simulink model "EarlyReturn12_2018a"  (R2018a)
settings: Solver=VariableStepAuto  StartTime=0.0  StopTime=0.1  RelTol=1e-3
settings Model: Creator=BEAR  LastModifiedBy=apple

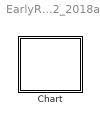
== system EarlyReturn12_2018a ==
  Chart : Stateflow chart  TreatAsAtomicUnit=on

== stateflow chart EarlyReturn12_2018a/Chart ==
  state A
    en: E;fprintf("enA_done")
  state B
    en: fprintf("enB")
  state C
    en: fprintf("enC")
  (default) -> A
  A -> B : E
  B -> C
  events: E local FUNCTION_CALL_EVENT
